simulink model "ForceControlInnerPositionLoop"  (R2020b)
settings: Solver=VariableStepAuto  StartTime=0.0  StopTime=0.6  RelTol=2.8421709430404007E-14
values from neighbouring files (symbols this model uses):
  K = diag([8 8 8 0.1 0.1 0.1])    [parameters.m]
  KD = diag([15 15 15])    [parameters.m]
  KFI = diag([1.5 1.5 1.5])    [parameters.m]
  KFP = diag([0.5 0.5 0.5])    [parameters.m]
  KP = diag([30 30 30])    [parameters.m]
  Md = 0.75*diag([1 1 1])    [parameters.m]
libraries: vrlib x1
settings Model: Creator=Edoardo  LastModifiedBy=Edoardo

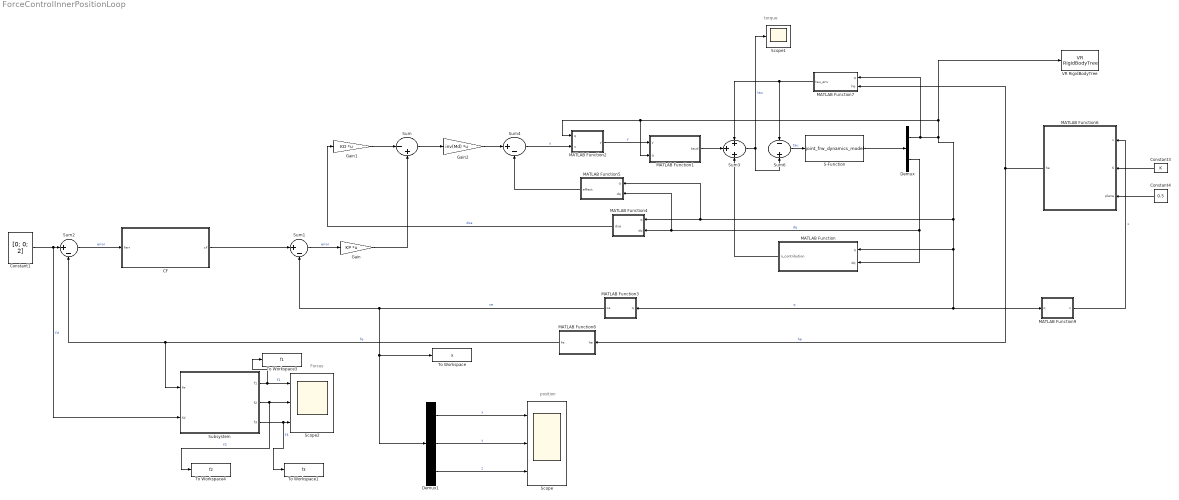
== system ForceControlInnerPositionLoop ==
  note: Forces
  note: torque
  note: position
  CF : Subsystem
  Constant1 : Constant  Value=[0; 0; 2]  VectorParams1D=off
  Constant3 : Constant  Value=K
  Constant4 : Constant  Value=0.5
  Demux : Demux  Outputs=2
  Demux1 : Demux  Outputs=3
  Gain : Gain  Gain=KP  Multiplication=Matrix(K*u) (u vector)
  Gain1 : Gain  Gain=KD  Multiplication=Matrix(K*u) (u vector)
  Gain2 : Gain  Gain=inv(Md)  Multiplication=Matrix(K*u) (u vector)
  MATLAB Function : MATLAB Function  TreatAsAtomicUnit=on
  MATLAB Function1 : MATLAB Function  TreatAsAtomicUnit=on
  MATLAB Function2 : MATLAB Function  TreatAsAtomicUnit=on
  MATLAB Function3 : MATLAB Function  TreatAsAtomicUnit=on
  MATLAB Function4 : MATLAB Function  TreatAsAtomicUnit=on
  MATLAB Function5 : MATLAB Function  TreatAsAtomicUnit=on
  MATLAB Function6 : MATLAB Function  TreatAsAtomicUnit=on
  MATLAB Function7 : MATLAB Function  TreatAsAtomicUnit=on
  MATLAB Function8 : MATLAB Function  TreatAsAtomicUnit=on
  MATLAB Function9 : MATLAB Function  TreatAsAtomicUnit=on
  S-Function : S-Function  FunctionName=joint_frw_dynamics_model  Parameters=myRobot  SFunctionDeploymentMode=off  EnableBusSupport=off
  Scope : Scope  NumInputPorts=3
  Scope1 : Scope
  Scope2 : Scope  NumInputPorts=3
  Subsystem : Subsystem
  Sum : Sum  Inputs=|-+
  Sum1 : Sum  Inputs=|+-
  Sum2 : Sum  Inputs=|+-
  Sum3 : Sum  Inputs=+++
  Sum4 : Sum  Inputs=|+-
  Sum6 : Sum  Inputs=-+
  To Workspace : ToWorkspace  VariableName=x  SaveFormat=Timeseries  SampleTime=-1
  To Workspace1 : ToWorkspace  VariableName=f3  SaveFormat=Timeseries  SampleTime=-1
  To Workspace3 : ToWorkspace  VariableName=f1  SaveFormat=Timeseries  SampleTime=-1
  To Workspace4 : ToWorkspace  VariableName=f2  SaveFormat=Timeseries  SampleTime=-1
  VR RigidBodyTree : vrlib/VR RigidBodyTree  RBT=robot  useRBT=on  Ts=-1  ForceViewerOpen=on
      settings: SourceProductBaseCode=SL
  wires:
  Sum1/1 -> Gain/1  "error"
  S-Function/1 -> Demux/1
  Sum3/1 -> Sum6/2, Scope1/1  "tau"
  Demux/2 -> MATLAB Function/2(dq), MATLAB Function4/2(dq), MATLAB Function5/2(dq)  "dq"
  Demux/1 -> MATLAB Function7/1(q), MATLAB Function4/1(q), MATLAB Function5/1(q), MATLAB Function9/1(q), MATLAB Function3/1(q), MATLAB Function/1(q), VR RigidBodyTree/1, MATLAB Function2/1(q), MATLAB Function1/2(q)  "q"
  MATLAB Function2/1(y) -> MATLAB Function1/1(y)  "y"
  MATLAB Function4/1(dxe) -> Gain1/1  "dxe"
  Demux1/1 -> Scope/1  "x"
  MATLAB Function3/1(xe) -> Demux1/1, To Workspace/1, Sum1/2  "xe"
  CF/1(xF) -> Sum1/1
  Constant4/1 -> MATLAB Function6/3(plane)
  Constant3/1 -> MATLAB Function6/2(K)
  MATLAB Function6/1(he) -> MATLAB Function7/2(he), MATLAB Function8/1(he)  "he"
  MATLAB Function/1(n_contribution) -> Sum3/3
  MATLAB Function1/1(taud) -> Sum3/2
  MATLAB Function7/1(tau_env) -> Sum6/1, Sum3/1
  Sum4/1 -> MATLAB Function2/2(u)  "u"
  MATLAB Function5/1(effect) -> Sum4/2
  Sum/1 -> Gain2/1
  Sum6/1 -> S-Function/1  "tau"
  Gain/1 -> Sum/2
  Gain1/1 -> Sum/1
  Constant1/1 -> Subsystem/2(fd), Sum2/1  "fd"
  Sum2/1 -> CF/1(ferr)  "error"
  Gain2/1 -> Sum4/1
  MATLAB Function8/1(fe) -> Sum2/2, Subsystem/1(fe)  "fe"
  MATLAB Function9/1(x) -> MATLAB Function6/1(x)  "x"
  Demux1/2 -> Scope/2  "y"
  Demux1/3 -> Scope/3  "z"
  Subsystem/1(f1) -> To Workspace3/1, Scope2/1  "f1"
  Subsystem/2(f2) -> To Workspace4/1, Scope2/2  "f2"
  Subsystem/3(f3) -> To Workspace1/1, Scope2/3  "f3"

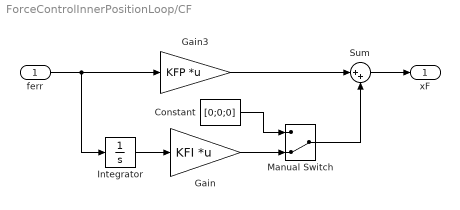
== system ForceControlInnerPositionLoop/CF ==
  ferr : Inport
  Constant : Constant  Value=[0;0;0]
  Gain : Gain  Gain=KFI  Multiplication=Matrix(K*u) (u vector)
  Gain3 : Gain  Gain=KFP  Multiplication=Matrix(K*u) (u vector)
  Integrator : Integrator
  Manual Switch : ManualSwitch  CurrentSetting=0
  Sum : Sum  Inputs=|++
  xF : Outport
  wires:
  ferr/1 -> Integrator/1, Gain3/1
  Gain3/1 -> Sum/1
  Sum/1 -> xF/1
  Integrator/1 -> Gain/1
  Gain/1 -> Manual Switch/2
  Manual Switch/1 -> Sum/2
  Constant/1 -> Manual Switch/1

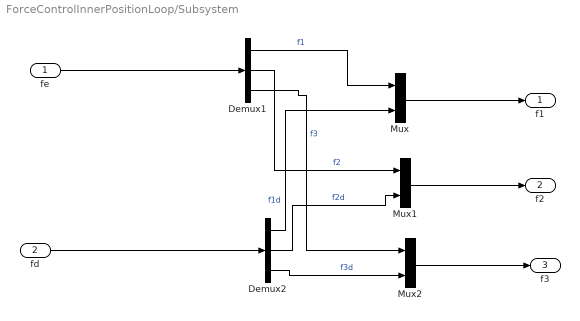
== system ForceControlInnerPositionLoop/Subsystem ==
  fe : Inport
  fd : Inport  Port=2
  Demux1 : Demux  Outputs=3
  Demux2 : Demux  Outputs=3
  Mux : Mux  Inputs=2
  Mux1 : Mux  Inputs=2
  Mux2 : Mux  Inputs=2
  f1 : Outport
  f2 : Outport  Port=2
  f3 : Outport  Port=3
  wires:
  Demux2/2 -> Mux1/2  "f2d"
  Mux2/1 -> f3/1
  Mux1/1 -> f2/1
  Demux2/1 -> Mux/2  "f1d"
  Demux1/2 -> Mux1/1  "f2"
  Demux1/1 -> Mux/1  "f1"
  Demux1/3 -> Mux2/1  "f3"
  Demux2/3 -> Mux2/2  "f3d"
  Mux/1 -> f1/1
  fe/1 -> Demux1/1
  fd/1 -> Demux2/1

== matlab function ForceControlInnerPositionLoop/MATLAB Function1 ==
  data: y input; taud output; q input size=3
function taud = B(y, q)

    taud = getBHatLagrangian(q)*y;

== matlab function ForceControlInnerPositionLoop/MATLAB Function ==
  data: q input size=3; n_contribution output; dq input size=3
function n_contribution = n(q,dq)
    n_contribution = getCHatLagrangian(q,dq)*dq + getGHatLagrangian(q);

== matlab function ForceControlInnerPositionLoop/MATLAB Function2 ==
  data: q input; u input; y output
function y = Jp_inv(q,u)

J = getJacobian(q);
Jp = J(1:3,:);

y =  pinv(Jp)*u;

== matlab function ForceControlInnerPositionLoop/MATLAB Function3 ==
  data: q input size=3; xe output size=3
function xe = Kp(q)

K = getDirectKinematics(q);

pos = K(1:3, 4);

xe = pos;

== matlab function ForceControlInnerPositionLoop/MATLAB Function4 ==
  data: q input size=3; dxe output size=3; dq input size=3
function dxe = Jp(q,dq)

J = getJacobian(q);
Jp = J(1:3,:);
dxe = Jp*dq;

== matlab function ForceControlInnerPositionLoop/MATLAB Function5 ==
  data: q input; effect output size=3; dq input
function effect = dJp(q, dq)

  dJa = getDAnalyticalJacobian(q, dq);
  dJap = dJa(1:3, 1:3);
  
  effect = dJap*dq;

== matlab function ForceControlInnerPositionLoop/MATLAB Function6 ==
  data: x input; he output; K input; plane input
function he = environment(x, K, plane)

% the robot is touching the environment 
if x(3) >= plane  % check is done in frame 0

    % set up the rest position frame
    xr = zeros(6,1);
    xr(3) = plane;
    
    % compute the forces

    xe = zeros(6,1);
    xe(3) = x(3);

    he = K * (xe - xr);
else
    % free motion
    he = zeros(6,1);
    
end

== matlab function ForceControlInnerPositionLoop/MATLAB Function7 ==
  data: q input; he input; tau_env output
function tau_env = JT(q, he)

tau_env = getJacobian(q)'*he;

== matlab function ForceControlInnerPositionLoop/MATLAB Function8 ==
  data: he input; fe output
function fe = he2fe(he)

fe = he(1:3);

== matlab function ForceControlInnerPositionLoop/MATLAB Function9 ==
  data: q input size=3; x output size=6
function x = K(q)

K = getDirectKinematics(q);

pos = K(1:3, 4);
rotm = K(1:3,1:3); 
ori = rotm2eul(rotm, 'ZYZ')';

x = [pos; ori];
